simulink model "MRAC"  (R2016b)
settings: Solver=ode45  StartTime=0.0  StopTime=4000  RelTol=1e-3  EnableMultiTasking=on
values from neighbouring files (symbols this model uses):
  tau = 2    [init.m]
  Td = 0.5    [init.m]
settings Model: Creator=Ibrahim  LastModifiedBy=DHC
settings DataIOCC: LimitDataPoints=on  SaveFormat=Array  SignalLoggingSaveFormat=ModelDataLogs
settings OptimizationCC: LifeSpan=inf
settings DebuggingCC: SolverPrmCheckMsg=warning  MultiTaskDSMMsg=warning  MultiTaskCondExecSysMsg=none  SFUnexpectedBacktrackingDiag=warning  SFNoUnconditionalDefaultTransitionDiag=warning  SFExecutionAtInitializationDiag=none
settings HardwareCC: ProdBitPerPointer=32  ProdBitPerSizeT=32  ProdBitPerPtrDiffT=32  ProdLargestAtomicFloat=None  ProdIntDivRoundTo=Undefined  ProdEndianess=Unspecified  ProdWordSize=32  ProdHWDeviceType=32-bit Generic
settings ModelReferenceCC: PropagateSignalLabelsOutOfModel=off
settings GRTTargetCC: TargetLangStandard=C89/C90 (ANSI)  GeneratePreprocessorConditionals=Disable all
settings ConfigComp: CovMetricSettings=dw  CovHtmlReporting=on  CovSaveCumulativeToWorkspaceVar=on  CovSaveSingleToWorkspaceVar=on  CovExternalEMLEnable=off  CovSFcnEnable=off

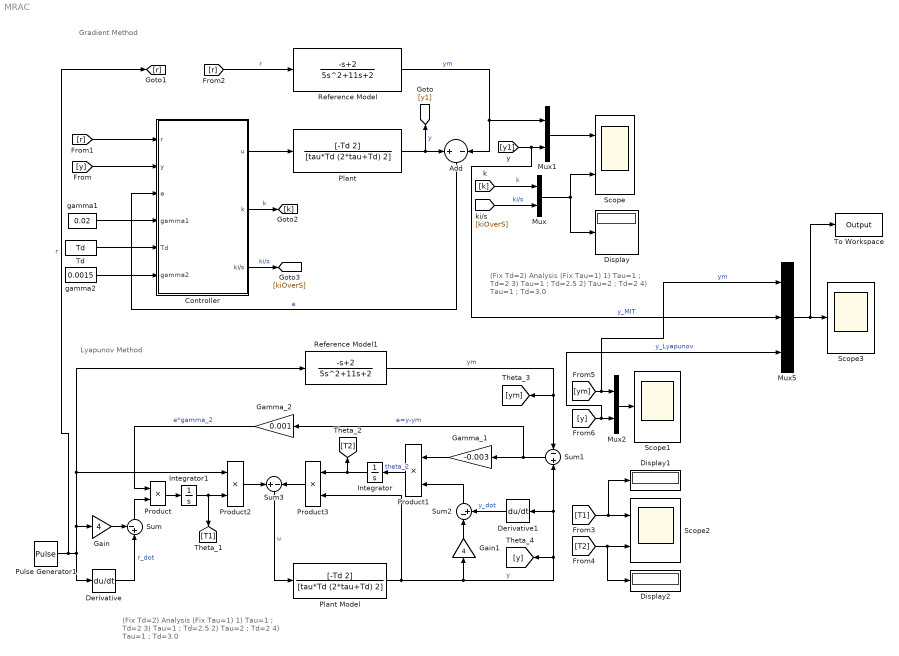
== system MRAC ==
  note: Gradient Method
  note: (Fix Td=2)    Analysis   (Fix Tau=1)
      | 1) Tau=1 ; Td=2        3) Tau=1 ; Td=2.5
      | 2) Tau=2 ; Td=2        4) Tau=1 ; Td=3.0
  note: Lyapunov Method
  note: (Fix Td=2)    Analysis   (Fix Tau=1)
      | 1) Tau=1 ; Td=2        3) Tau=1 ; Td=2.5
      | 2) Tau=2 ; Td=2        4) Tau=1 ; Td=3.0
  Add : Sum  Inputs=+|-
  Controller : Subsystem
  Derivative : Derivative
  Derivative1 : Derivative
  Display : Display
  Display1 : Display
  Display2 : Display
  Gain : Gain  Gain=4
  Gain1 : Gain  Gain=4
  Gamma_1 : Gain  Gain=-0.003
  Gamma_2 : Gain  Gain=0.001
  Integrator : Integrator
  Integrator1 : Integrator
  Mux : Mux  Inputs=2
  Mux1 : Mux  Inputs=2
  Mux2 : Mux  Inputs=2
  Mux5 : Mux  Inputs=3
  Plant : TransferFcn  Numerator=[-Td 2]  Denominator=[tau*Td (2*tau+Td) 2]
  Plant Model : TransferFcn  Numerator=[-Td 2]  Denominator=[tau*Td (2*tau+Td) 2]
  Product{,1..3} (4 alike) : Product
  Pulse Generator1 : DiscretePulseGenerator  PulseType=Time based  Amplitude=3.5  Period=1200  PulseWidth=80
  Reference Model : TransferFcn  Numerator=[-1 2]  Denominator=[5 11 2]
  Reference Model1 : TransferFcn  Numerator=[-1 2]  Denominator=[5 11 2]
  Scope : Scope  NumInputPorts=2
  Scope1 : Scope
  Scope2 : Scope  NumInputPorts=2
  Scope3 : Scope
  Sum : Sum  Inputs=-+|
  Sum1 : Sum  Inputs=-|+
  Sum2 : Sum  Inputs=|-+
  Sum3 : Sum  Inputs=+|-
  Td : Constant  Value=Td
  To Workspace : ToWorkspace  VariableName=Output  SaveFormat=Timeseries  SampleTime=-1
  gamma1 : Constant  Value=0.02
  gamma2 : Constant  Value=0.0015
  wires:
  Reference Model/1 -> Add/2, Mux1/1  "ym"
  Plant/1 -> [y1], Add/1  "y"
  Controller/1(u) -> Plant/1
  [y] -> Controller/2(y)
  [r] -> Controller/1(r)
  Add/1 -> Controller/3(e)  "e"
  [r] -> Reference Model/1  "r"
  gamma1/1 -> Controller/4(gamma1)
  Controller/2(k) -> [k]  "k"
  Controller/3(ki/s) -> [kiOverS]  "ki/s"
  Mux/1 -> Display/1, Scope/2
  [k] -> Mux/1  "k"
  [kiOverS] -> Mux/2  "ki/s"
  Mux1/1 -> Scope/1
  gamma2/1 -> Controller/6(gamma2)
  Td/1 -> Controller/5(Td)
  Plant Model/1 -> Gain1/1, [y], Sum1/2, Derivative1/1, Product3/2  "y"
  Sum1/1 -> Gamma_2/1, Gamma_1/1  "e=y-ym"
  Pulse Generator1/1 -> [r], Derivative/1, Gain/1, Reference Model1/1, Product2/1  "r"
  Gain/1 -> Sum/1
  Gamma_2/1 -> Product/1  "e*gamma_2"
  Sum/1 -> Product/2
  Derivative1/1 -> Sum2/2  "y_dot"
  Sum2/1 -> Product1/2
  Product1/1 -> Integrator/1  "theta_2"
  Product2/1 -> Sum3/1
  Sum3/1 -> Plant Model/1  "u"
  [T1] -> Display1/1, Scope2/1
  [T2] -> Display2/1, Scope2/2
  [y] -> Mux5/3, Mux2/2  "y_Lyapunov"
  Mux2/1 -> Scope1/1
  Product/1 -> Integrator1/1
  Gamma_1/1 -> Product1/1
  Gain1/1 -> Sum2/1
  Product3/1 -> Sum3/2
  Derivative/1 -> Sum/2  "r_dot"
  Integrator/1 -> Product3/1, [T2]
  Integrator1/1 -> [T1], Product2/2
  Reference Model1/1 -> [ym], Sum1/1  "ym"
  [ym] -> Mux5/1, Mux2/1  "ym"
  [y1] -> Mux5/2, Mux1/2  "y_MIT"
  Mux5/1 -> To Workspace/1, Scope3/1

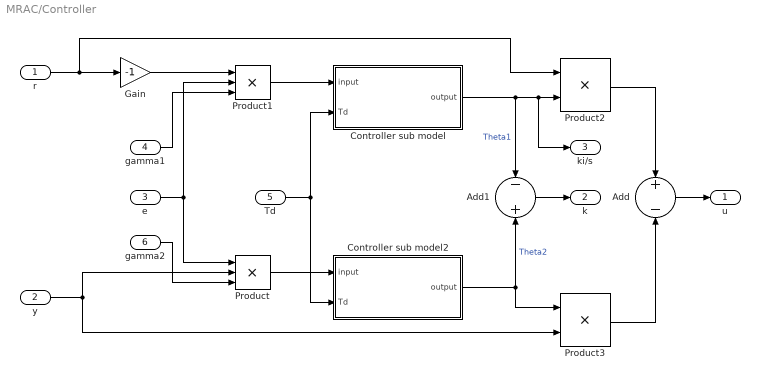
== system MRAC/Controller ==
  r : Inport
  y : Inport  Port=2
  e : Inport  Port=3
  gamma1 : Inport  Port=4
  Td : Inport  Port=5
  gamma2 : Inport  Port=6
  Add : Sum  Inputs=+-
  Add1 : Sum  Inputs=-+
  Controller sub model : Subsystem
  Controller sub model2 : Subsystem
  Gain : Gain  Gain=-1
  Product : Product  Inputs=3  InputSameDT=on
  Product1 : Product  Inputs=3  InputSameDT=on
  Product2 : Product  InputSameDT=on
  Product3 : Product  InputSameDT=on
  u : Outport
  k : Outport  Port=2
  ki/s : Outport  Port=3
  wires:
  e/1 -> Product1/2, Product/1
  r/1 -> Product2/1, Gain/1
  Product/1 -> Controller sub model2/1(input)
  Product1/1 -> Controller sub model/1(input)
  y/1 -> Product3/2, Product/2
  Gain/1 -> Product1/1
  Controller sub model/1(output) -> Add1/1, ki/s/1, Product2/2  "Theta1"
  Controller sub model2/1(output) -> Product3/1, Add1/2  "Theta2"
  Add/1 -> u/1
  Product2/1 -> Add/1
  Product3/1 -> Add/2
  Add1/1 -> k/1
  Td/1 -> Controller sub model/2(Td), Controller sub model2/2(Td)
  gamma1/1 -> Product1/3
  gamma2/1 -> Product/3

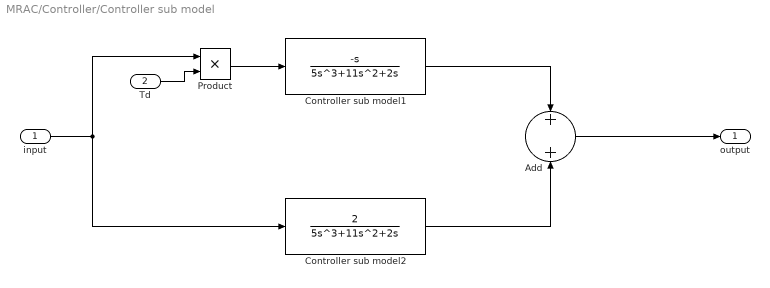
== system MRAC/Controller/Controller sub model ==
  input : Inport
  Td : Inport  Port=2
  Add : Sum
  Controller sub model1 : TransferFcn  Numerator=[-1 0]  Denominator=[5 11 2 0]
  Controller sub model2 : TransferFcn  Numerator=[2]  Denominator=[5 11 2 0]
  Product : Product
  output : Outport
  wires:
  Product/1 -> Controller sub model1/1
  Td/1 -> Product/2
  Controller sub model1/1 -> Add/1
  Controller sub model2/1 -> Add/2
  Add/1 -> output/1
  input/1 -> Controller sub model2/1, Product/1

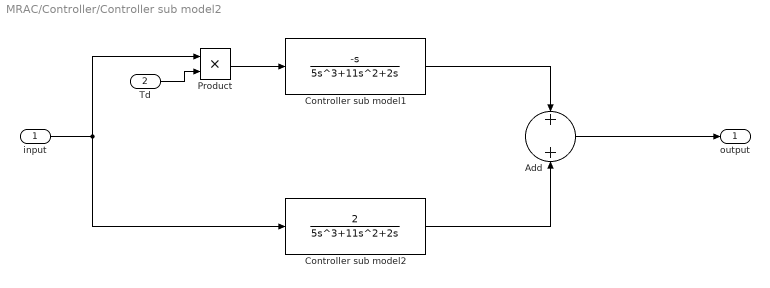
== system MRAC/Controller/Controller sub model2 ==
  input : Inport
  Td : Inport  Port=2
  Add : Sum
  Controller sub model1 : TransferFcn  Numerator=[-1 0]  Denominator=[5 11 2 0]
  Controller sub model2 : TransferFcn  Numerator=[2]  Denominator=[5 11 2 0]
  Product : Product
  output : Outport
  wires:
  Product/1 -> Controller sub model1/1
  Td/1 -> Product/2
  Controller sub model1/1 -> Add/1
  Controller sub model2/1 -> Add/2
  Add/1 -> output/1
  input/1 -> Controller sub model2/1, Product/1
